simulink model "sema"  (R2025b)
settings: Solver=VariableStepAuto  StartTime=0.0  StopTime=160  RelTol=1e-3
libraries: fuzblock x1, simulink_extras x1
settings Model: Creator=PC  LastModifiedBy=urosp

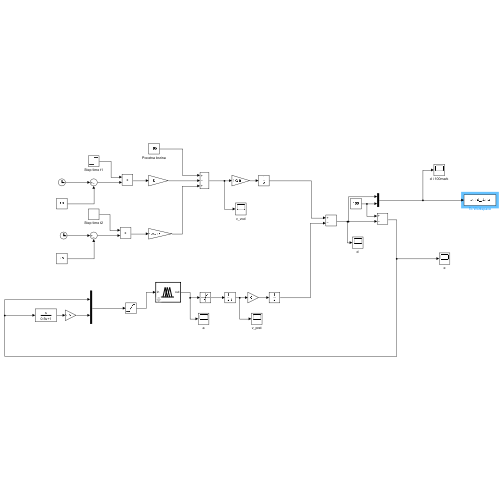
[thumbnail: Simulink's stored preview of the top-level diagram]
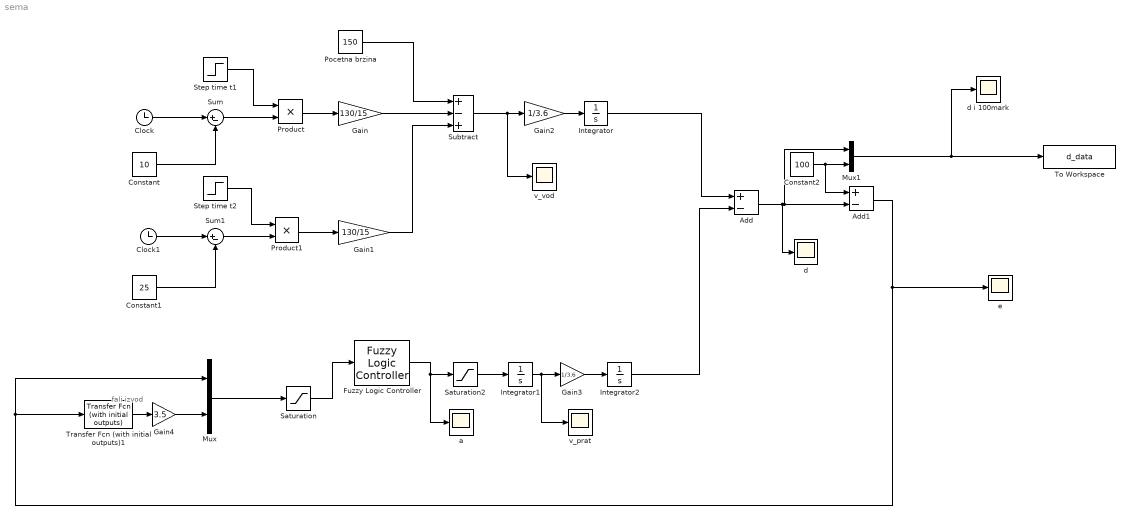
== system sema ==
  note: fali
      |  izvod
  Add : Sum  Inputs=+-
  Add1 : Sum  Inputs=+-
  Clock : Clock
  Clock1 : Clock
      settings: Decimation=25
  Constant : Constant  Value=10
  Constant1 : Constant  Value=25
  Constant2 : Constant  Value=100
  Fuzzy Logic Controller : fuzblock/Fuzzy Logic  Controller  FIS='Zadatak.fis'  OutputSampleNumber=101  DataType=double  UseLookupTable=off  NumBreakpoints=10  FuzzifiedInputs=off  RuleFiringStrengths=off  RuleOutputs=off  AggregatedOutputs=off  SimulateUsing=Interpreted execution  OutOfRangeInputValueMessage=warning  NoRuleFiredMessage=warning  EmptyOutputFuzzySetMessage=warning
  Gain : Gain  Gain=130/15
  Gain1 : Gain  Gain=130/15
  Gain2 : Gain  Gain=1/3.6
  Gain3 : Gain  Gain=1/3.6
  Gain4 : Gain  Gain=3.5
  Integrator : Integrator  InitialCondition=70
  Integrator1 : Integrator  InitialCondition=120  LimitOutput=on  LowerSaturationLimit=0
  Integrator2 : Integrator
  Mux : Mux  Inputs=2
  Mux1 : Mux  Inputs=2
  Pocetna brzina : Constant  Value=150
  Product : Product
  Product1 : Product
  Saturation : Saturate  UpperLimit=100  LowerLimit=-100
  Saturation2 : Saturate  UpperLimit=10  LowerLimit=-10
  Step time t1 : Step  Time=10  SampleTime=0
  Step time t2 : Step  Time=25  SampleTime=0
  Subtract : Sum  Inputs=+-+
  Sum : Sum  Inputs=|+-
  Sum1 : Sum  Inputs=|+-
  To Workspace : ToWorkspace  VariableName=d_data  SaveFormat=Structure With Time  SampleTime=-1
      settings: MaxDataPoints=200
  Transfer Fcn (with initial outputs)1 : simulink_extras/Additional Linear/Transfer Fcn (with initial outputs)  N=[1 0]  D="[0.5  1]"  Y0=.00000001  U0=0
  a : Scope
      settings: ActiveDisplayYMinimum=-10.80693457204373  ActiveDisplayYMaximum=5.2766890788433649  DataLoggingVariableName=ScopeData2
  d : Scope
      settings: ActiveDisplayYMinimum=-23.703880297757181  ActiveDisplayYMaximum=190.13518842865145  DataLoggingVariableName=ScopeData2
  d i 100mark : Scope
      settings: ActiveDisplayYMinimum=-103.07264614637774  ActiveDisplayYMaximum=539.07416804469767
  e : Scope
      settings: ActiveDisplayYMinimum=-25.2230253712219  ActiveDisplayYMaximum=76.556720821809336
  v_prat : Scope
      settings: ActiveDisplayYMinimum=41.8836748172326  ActiveDisplayYMaximum=196.75283100000792  DataLoggingVariableName=ScopeData3
  v_vod : Scope
      settings: ActiveDisplayYMinimum=1.9500840147389908  ActiveDisplayYMaximum=204.91263566031472
  wires:
  Clock/1 -> Sum/1
  Constant/1 -> Sum/2
  Clock1/1 -> Sum1/1
  Constant1/1 -> Sum1/2
  Sum/1 -> Product/2
  Sum1/1 -> Product1/2
  Step time t2/1 -> Product1/1
  Step time t1/1 -> Product/1
  Product1/1 -> Gain1/1
  Product/1 -> Gain/1
  Pocetna brzina/1 -> Subtract/1
  Gain/1 -> Subtract/2
  Gain1/1 -> Subtract/3
  Subtract/1 -> Gain2/1, v_vod/1
  Gain2/1 -> Integrator/1
  Fuzzy Logic Controller/1 -> a/1, Saturation2/1
  Integrator2/1 -> Add/2
  Add/1 -> d/1, Mux1/1, Add1/2
  Constant2/1 -> Add1/1, Mux1/2
  Mux1/1 -> To Workspace/1, d i 100mark/1
  Add1/1 -> e/1, Transfer Fcn (with initial outputs)1/1, Mux/1
  Gain3/1 -> Integrator2/1
  Saturation2/1 -> Integrator1/1
  Integrator/1 -> Add/1
  Mux/1 -> Saturation/1
  Saturation/1 -> Fuzzy Logic Controller/1
  Integrator1/1 -> v_prat/1, Gain3/1
  Transfer Fcn (with initial outputs)1/1 -> Gain4/1
  Gain4/1 -> Mux/2
